simulink model "test4"  (R2015a)
settings: Solver=ode3  SolverMode=SingleTasking  StartTime=0.0  StopTime=10.0  RelTol=1e-3
libraries: simulink_extras x1, simulink x1
settings Model: ExtModeTrigDuration=2  Creator=kkhoo  LastModifiedBy=kkhoo
settings OptimizationCC: OptimizeModelRefInitCode=on  LifeSpan=1
settings DebuggingCC: UnderspecifiedInitializationDetection=Classic  MergeDetectMultiDrivingBlocksExec=none
settings HardwareCC: ProdBitPerInt=16  ProdBitPerPointer=8  ProdIntDivRoundTo=Zero  ProdEndianess=LittleEndian  ProdWordSize=8  ProdHWDeviceType=Atmel->AVR
settings RTWCC: SystemTargetFile=realtime.tlc  GenerateMakefile=off  TemplateMakefile=realtime.tmf  Description=Run on Target Hardware  RTWVerbose=off  CustomSource=src/Engduino.h src/engduino_wrappers.cpp
settings ERTTargetCC: CombineOutputUpdateFcns=off  ExtModeTransport=3  ExtModeMexFile=ext_serial_win32_comm_rtt  ExtModeMexArgs=0 1 9600  ERTSrcFileBannerTemplate=realtime_code_template.cgt  ERTHdrFileBannerTemplate=realtime_code_template.cgt  ERTDataSrcFileTemplate=realtime_code_template.cgt  ERTDataHdrFileTemplate=realtime_code_template.cgt  ERTCustomFileTemplate=realtime_file_process.tlc

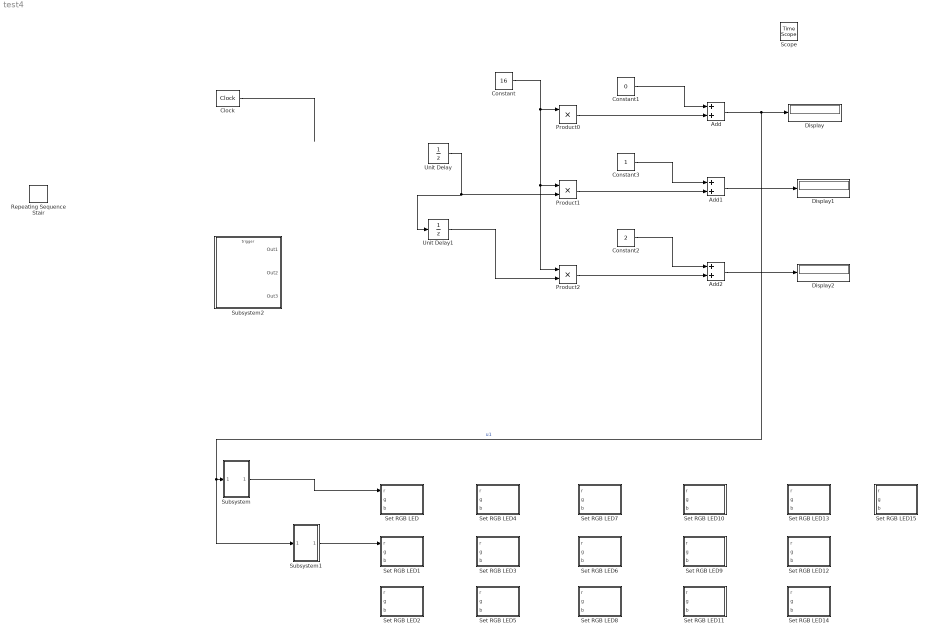
== system test4 ==
  Add : Sum  AccumDataTypeStr=single
  Add1 : Sum  AccumDataTypeStr=single
  Add2 : Sum  AccumDataTypeStr=single
  Clock : simulink_extras/Flip Flops/Clock  period=1000000
  Constant : Constant  Value=16  OutDataTypeStr=single
  Constant1 : Constant  Value=0  OutDataTypeStr=single
  Constant2 : Constant  Value=2  OutDataTypeStr=single
  Constant3 : Constant  OutDataTypeStr=single
  Display : Display
  Display1 : Display
  Display2 : Display
  "Product0 " : Product  OutDataTypeStr=single
  Product1 : Product  OutDataTypeStr=single
  Product2 : Product  OutDataTypeStr=single  InputSameDT=on
  Repeating Sequence Stair : simulink/Sources/Repeating Sequence Stair  OutValues=[0 1 2 3 4 5 6 7 8 9 10 11 12 13 14 15].'  tsamp=0.001  OutMin=[]  OutMax=[]  OutDataTypeStr=single  OutputDataTypeScalingMode=single  OutDataType=fixdt(0,8)  ConRadixGroup=Best Precision: Vector-wise  OutScaling=2^-12
  Scope : TimeScope
  Set RGB LED : MATLAB Function  LoadFcn=|  TreatAsAtomicUnit=on  mask(RGB LED){led_index=0}
      | set_param(gcs, 'CustomSource', strjoin(unique([strsplit(get_param(gcs, 'CustomSource')) ...
      |  'src/engduino_wrappers.cpp' 'src/Engduino.h'])));
      mask prompts: led_index "LED index"
      mask help:
      | Control the Red, Green and Blue color values of the LED specified by the LED index parameter.
      | Both the LED index and the three color values are of type uint8 and must be in the range 0-15.
      settings: AttributesFormatString=LED %<led_index>
  Set RGB LED1 : MATLAB Function  LoadFcn=|  TreatAsAtomicUnit=on  mask(RGB LED){led_index=1}
      | set_param(gcs, 'CustomSource', strjoin(unique([strsplit(get_param(gcs, 'CustomSource')) ...
      |  'src/engduino_wrappers.cpp' 'src/Engduino.h'])));
      mask prompts: led_index "LED index"
      mask help:
      | Control the Red, Green and Blue color values of the LED specified by the LED index parameter.
      | Both the LED index and the three color values are of type uint8 and must be in the range 0-15.
      settings: AttributesFormatString=LED %<led_index>
  Set RGB LED10 : MATLAB Function  LoadFcn=|  TreatAsAtomicUnit=on  mask(RGB LED){led_index=9}
      | set_param(gcs, 'CustomSource', strjoin(unique([strsplit(get_param(gcs, 'CustomSource')) ...
      |  'src/engduino_wrappers.cpp' 'src/Engduino.h'])));
      mask prompts: led_index "LED index"
      mask help:
      | Control the Red, Green and Blue color values of the LED specified by the LED index parameter.
      | Both the LED index and the three color values are of type uint8 and must be in the range 0-15.
      settings: AttributesFormatString=LED %<led_index>
  Set RGB LED11 : MATLAB Function  LoadFcn=|  TreatAsAtomicUnit=on  mask(RGB LED){led_index=11}
      | set_param(gcs, 'CustomSource', strjoin(unique([strsplit(get_param(gcs, 'CustomSource')) ...
      |  'src/engduino_wrappers.cpp' 'src/Engduino.h'])));
      mask prompts: led_index "LED index"
      mask help:
      | Control the Red, Green and Blue color values of the LED specified by the LED index parameter.
      | Both the LED index and the three color values are of type uint8 and must be in the range 0-15.
      settings: AttributesFormatString=LED %<led_index>
  Set RGB LED12 : MATLAB Function  LoadFcn=|  TreatAsAtomicUnit=on  mask(RGB LED){led_index=13}
      | set_param(gcs, 'CustomSource', strjoin(unique([strsplit(get_param(gcs, 'CustomSource')) ...
      |  'src/engduino_wrappers.cpp' 'src/Engduino.h'])));
      mask prompts: led_index "LED index"
      mask help:
      | Control the Red, Green and Blue color values of the LED specified by the LED index parameter.
      | Both the LED index and the three color values are of type uint8 and must be in the range 0-15.
      settings: AttributesFormatString=LED %<led_index>
  Set RGB LED13 : MATLAB Function  LoadFcn=|  TreatAsAtomicUnit=on  mask(RGB LED){led_index=12}
      | set_param(gcs, 'CustomSource', strjoin(unique([strsplit(get_param(gcs, 'CustomSource')) ...
      |  'src/engduino_wrappers.cpp' 'src/Engduino.h'])));
      mask prompts: led_index "LED index"
      mask help:
      | Control the Red, Green and Blue color values of the LED specified by the LED index parameter.
      | Both the LED index and the three color values are of type uint8 and must be in the range 0-15.
      settings: AttributesFormatString=LED %<led_index>
  Set RGB LED14 : MATLAB Function  LoadFcn=|  TreatAsAtomicUnit=on  mask(RGB LED){led_index=14}
      | set_param(gcs, 'CustomSource', strjoin(unique([strsplit(get_param(gcs, 'CustomSource')) ...
      |  'src/engduino_wrappers.cpp' 'src/Engduino.h'])));
      mask prompts: led_index "LED index"
      mask help:
      | Control the Red, Green and Blue color values of the LED specified by the LED index parameter.
      | Both the LED index and the three color values are of type uint8 and must be in the range 0-15.
      settings: AttributesFormatString=LED %<led_index>
  Set RGB LED15 : MATLAB Function  LoadFcn=|  TreatAsAtomicUnit=on  mask(RGB LED){led_index=15}
      | set_param(gcs, 'CustomSource', strjoin(unique([strsplit(get_param(gcs, 'CustomSource')) ...
      |  'src/engduino_wrappers.cpp' 'src/Engduino.h'])));
      mask prompts: led_index "LED index"
      mask help:
      | Control the Red, Green and Blue color values of the LED specified by the LED index parameter.
      | Both the LED index and the three color values are of type uint8 and must be in the range 0-15.
      settings: AttributesFormatString=LED %<led_index>
  Set RGB LED2 : MATLAB Function  LoadFcn=|  TreatAsAtomicUnit=on  mask(RGB LED){led_index=2}
      | set_param(gcs, 'CustomSource', strjoin(unique([strsplit(get_param(gcs, 'CustomSource')) ...
      |  'src/engduino_wrappers.cpp' 'src/Engduino.h'])));
      mask prompts: led_index "LED index"
      mask help:
      | Control the Red, Green and Blue color values of the LED specified by the LED index parameter.
      | Both the LED index and the three color values are of type uint8 and must be in the range 0-15.
      settings: AttributesFormatString=LED %<led_index>
  Set RGB LED3 : MATLAB Function  LoadFcn=|  TreatAsAtomicUnit=on  mask(RGB LED){led_index=4}
      | set_param(gcs, 'CustomSource', strjoin(unique([strsplit(get_param(gcs, 'CustomSource')) ...
      |  'src/engduino_wrappers.cpp' 'src/Engduino.h'])));
      mask prompts: led_index "LED index"
      mask help:
      | Control the Red, Green and Blue color values of the LED specified by the LED index parameter.
      | Both the LED index and the three color values are of type uint8 and must be in the range 0-15.
      settings: AttributesFormatString=LED %<led_index>
  Set RGB LED4 : MATLAB Function  LoadFcn=|  TreatAsAtomicUnit=on  mask(RGB LED){led_index=3}
      | set_param(gcs, 'CustomSource', strjoin(unique([strsplit(get_param(gcs, 'CustomSource')) ...
      |  'src/engduino_wrappers.cpp' 'src/Engduino.h'])));
      mask prompts: led_index "LED index"
      mask help:
      | Control the Red, Green and Blue color values of the LED specified by the LED index parameter.
      | Both the LED index and the three color values are of type uint8 and must be in the range 0-15.
      settings: AttributesFormatString=LED %<led_index>
  Set RGB LED5 : MATLAB Function  LoadFcn=|  TreatAsAtomicUnit=on  mask(RGB LED){led_index=5}
      | set_param(gcs, 'CustomSource', strjoin(unique([strsplit(get_param(gcs, 'CustomSource')) ...
      |  'src/engduino_wrappers.cpp' 'src/Engduino.h'])));
      mask prompts: led_index "LED index"
      mask help:
      | Control the Red, Green and Blue color values of the LED specified by the LED index parameter.
      | Both the LED index and the three color values are of type uint8 and must be in the range 0-15.
      settings: AttributesFormatString=LED %<led_index>
  Set RGB LED6 : MATLAB Function  LoadFcn=|  TreatAsAtomicUnit=on  mask(RGB LED){led_index=7}
      | set_param(gcs, 'CustomSource', strjoin(unique([strsplit(get_param(gcs, 'CustomSource')) ...
      |  'src/engduino_wrappers.cpp' 'src/Engduino.h'])));
      mask prompts: led_index "LED index"
      mask help:
      | Control the Red, Green and Blue color values of the LED specified by the LED index parameter.
      | Both the LED index and the three color values are of type uint8 and must be in the range 0-15.
      settings: AttributesFormatString=LED %<led_index>
  Set RGB LED7 : MATLAB Function  LoadFcn=|  TreatAsAtomicUnit=on  mask(RGB LED){led_index=6}
      | set_param(gcs, 'CustomSource', strjoin(unique([strsplit(get_param(gcs, 'CustomSource')) ...
      |  'src/engduino_wrappers.cpp' 'src/Engduino.h'])));
      mask prompts: led_index "LED index"
      mask help:
      | Control the Red, Green and Blue color values of the LED specified by the LED index parameter.
      | Both the LED index and the three color values are of type uint8 and must be in the range 0-15.
      settings: AttributesFormatString=LED %<led_index>
  Set RGB LED8 : MATLAB Function  LoadFcn=|  TreatAsAtomicUnit=on  mask(RGB LED){led_index=8}
      | set_param(gcs, 'CustomSource', strjoin(unique([strsplit(get_param(gcs, 'CustomSource')) ...
      |  'src/engduino_wrappers.cpp' 'src/Engduino.h'])));
      mask prompts: led_index "LED index"
      mask help:
      | Control the Red, Green and Blue color values of the LED specified by the LED index parameter.
      | Both the LED index and the three color values are of type uint8 and must be in the range 0-15.
      settings: AttributesFormatString=LED %<led_index>
  Set RGB LED9 : MATLAB Function  LoadFcn=|  TreatAsAtomicUnit=on  mask(RGB LED){led_index=10}
      | set_param(gcs, 'CustomSource', strjoin(unique([strsplit(get_param(gcs, 'CustomSource')) ...
      |  'src/engduino_wrappers.cpp' 'src/Engduino.h'])));
      mask prompts: led_index "LED index"
      mask help:
      | Control the Red, Green and Blue color values of the LED specified by the LED index parameter.
      | Both the LED index and the three color values are of type uint8 and must be in the range 0-15.
      settings: AttributesFormatString=LED %<led_index>
  Subsystem : Subsystem
  Subsystem1 : Subsystem
  Subsystem2 : Subsystem
  Unit Delay : UnitDelay  SampleTime=-1
  Unit Delay1 : UnitDelay  SampleTime=-1
  wires:
  Unit Delay/1 -> Unit Delay1/1, Product1/2
  Constant/1 -> "Product0 "/1, Product2/1, Product1/1
  Unit Delay1/1 -> Product2/2
  Constant1/1 -> Add/1
  "Product0 "/1 -> Add/2
  Constant3/1 -> Add1/1
  Product1/1 -> Add1/2
  Constant2/1 -> Add2/1
  Product2/1 -> Add2/2
  Add/1 -> Subsystem1/1(In1), Subsystem/1(In1), Display/1  "u1"
  Add1/1 -> Display1/1
  Add2/1 -> Display2/1
  Subsystem/1(Out1) -> Set RGB LED/1(r)
  Subsystem1/1(Out1) -> Set RGB LED1/1(r)
  ? -> Scope/1, "Product0 "/2, Unit Delay/1
  Clock/1 -> ?

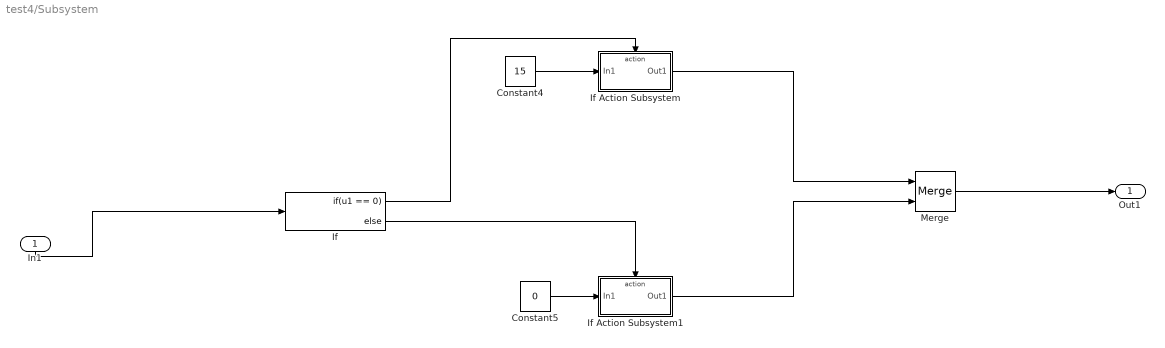
== system test4/Subsystem ==
  In1 : Inport
  Constant4 : Constant  Value=15  OutDataTypeStr=uint8
  Constant5 : Constant  Value=0  OutDataTypeStr=uint8
  If : If  IfExpression=u1 == 0
  If Action Subsystem : Subsystem  TreatAsAtomicUnit=on
  If Action Subsystem1 : Subsystem  TreatAsAtomicUnit=on
  Merge : Merge
  Out1 : Outport  OutDataTypeStr=uint8
  wires:
  If/1 -> If Action Subsystem/Action
  If/2 -> If Action Subsystem1/Action
  In1/1 -> If/1
  Constant5/1 -> If Action Subsystem1/1(In1)
  Merge/1 -> Out1/1
  Constant4/1 -> If Action Subsystem/1(In1)
  If Action Subsystem/1(Out1) -> Merge/1
  If Action Subsystem1/1(Out1) -> Merge/2

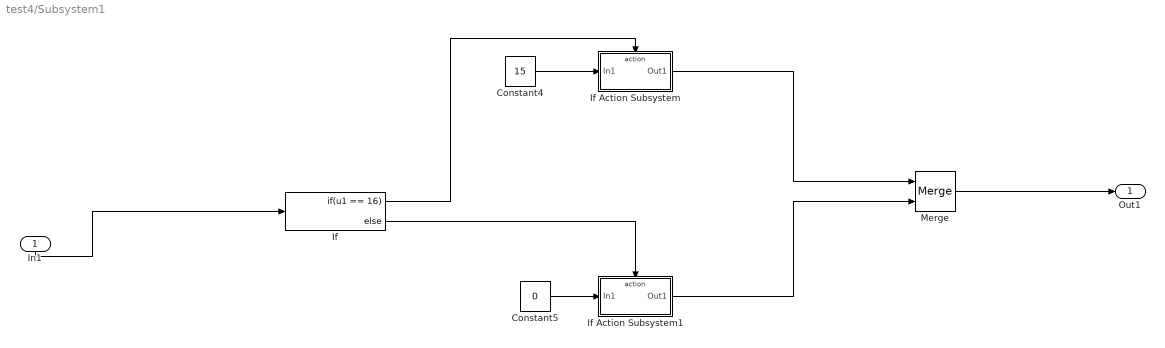
== system test4/Subsystem1 ==
  In1 : Inport
  Constant4 : Constant  Value=15  OutDataTypeStr=uint8
  Constant5 : Constant  Value=0  OutDataTypeStr=uint8
  If : If  IfExpression=u1 == 16
  If Action Subsystem : Subsystem  TreatAsAtomicUnit=on
  If Action Subsystem1 : Subsystem  TreatAsAtomicUnit=on
  Merge : Merge
  Out1 : Outport  OutDataTypeStr=uint8
  wires:
  If/1 -> If Action Subsystem/Action
  If/2 -> If Action Subsystem1/Action
  In1/1 -> If/1
  Constant5/1 -> If Action Subsystem1/1(In1)
  Merge/1 -> Out1/1
  Constant4/1 -> If Action Subsystem/1(In1)
  If Action Subsystem/1(Out1) -> Merge/1
  If Action Subsystem1/1(Out1) -> Merge/2

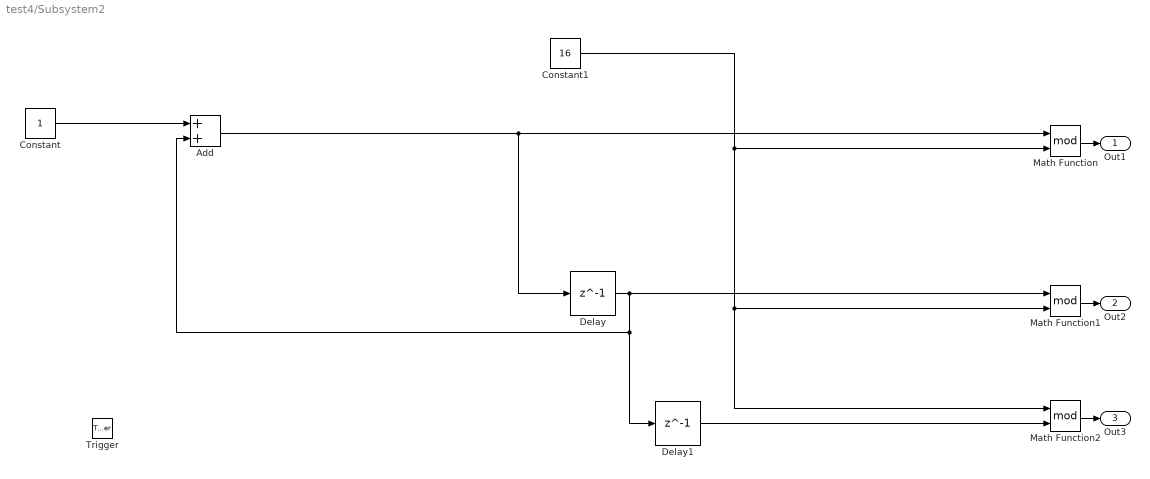
== system test4/Subsystem2 ==
  Trigger : TriggerPort  PortDimensions=1
  Add : Sum
  Constant : Constant
  Constant1 : Constant  Value=16
  Delay : Delay  DelayLength=1  InitialCondition=0
  Delay1 : Delay  DelayLength=1  InitialCondition=0
  Math Function : Math  Operator=mod  SaturateOnIntegerOverflow=on
  Math Function1 : Math  Operator=mod  SaturateOnIntegerOverflow=on
  Math Function2 : Math  Operator=mod  SaturateOnIntegerOverflow=on
  Out1 : Outport
  Out2 : Outport  Port=2
  Out3 : Outport  Port=3
  wires:
  Add/1 -> Math Function/1, Delay/1
  Constant/1 -> Add/1
  Math Function/1 -> Out1/1
  Math Function2/1 -> Out3/1
  Delay1/1 -> Math Function2/2
  Math Function1/1 -> Out2/1
  Constant1/1 -> Math Function/2, Math Function2/1, Math Function1/2
  Delay/1 -> Delay1/1, Add/2, Math Function1/1

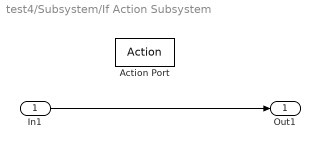
== system test4/Subsystem/If Action Subsystem ==
  In1 : Inport
  Action Port : ActionPort  ActionType=then
  Out1 : Outport  OutDataTypeStr=uint8
  wires:
  In1/1 -> Out1/1

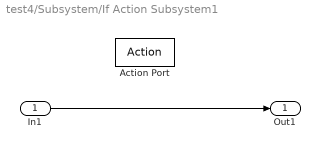
== system test4/Subsystem/If Action Subsystem1 ==
  In1 : Inport
  Action Port : ActionPort  ActionType=else
  Out1 : Outport  OutDataTypeStr=uint8
  wires:
  In1/1 -> Out1/1

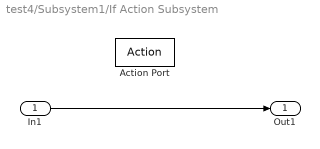
== system test4/Subsystem1/If Action Subsystem ==
  In1 : Inport
  Action Port : ActionPort  ActionType=then
  Out1 : Outport  OutDataTypeStr=uint8
  wires:
  In1/1 -> Out1/1

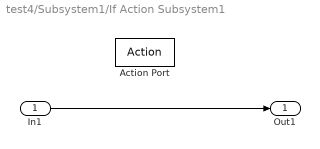
== system test4/Subsystem1/If Action Subsystem1 ==
  In1 : Inport
  Action Port : ActionPort  ActionType=else
  Out1 : Outport  OutDataTypeStr=uint8
  wires:
  In1/1 -> Out1/1

== matlab function test4/Set RGB LED2 ==
  data: led_index parameter uint8 [0..15]; r input uint8 [0..15]; g input uint8 [0..15]; b input uint8 [0..15]
function rgb_led(led_index, r, g, b)

if strcmp(coder.target, 'rtw')
    coder.ceval('rgb_leds_wrapper', led_index, r, g, b);
end

== matlab function test4/Set RGB LED3 ==
  data: led_index parameter uint8 [0..15]; r input uint8 [0..15]; g input uint8 [0..15]; b input uint8 [0..15]
function rgb_led(led_index, r, g, b)

if strcmp(coder.target, 'rtw')
    coder.ceval('rgb_leds_wrapper', led_index, r, g, b);
end

== matlab function test4/Set RGB LED ==
  data: led_index parameter uint8 [0..15]; r input uint8 [0..15]; g input uint8 [0..15]; b input uint8 [0..15]
function rgb_led(led_index, r, g, b)

if strcmp(coder.target, 'rtw')
    coder.ceval('rgb_leds_wrapper', led_index, r, g, b);
end

== matlab function test4/Set RGB LED1 ==
  data: led_index parameter uint8 [0..15]; r input uint8 [0..15]; g input uint8 [0..15]; b input uint8 [0..15]
function rgb_led(led_index, r, g, b)

if strcmp(coder.target, 'rtw')
    coder.ceval('rgb_leds_wrapper', led_index, r, g, b);
end

== matlab function test4/Set RGB LED4 ==
  data: led_index parameter uint8 [0..15]; r input uint8 [0..15]; g input uint8 [0..15]; b input uint8 [0..15]
function rgb_led(led_index, r, g, b)

if strcmp(coder.target, 'rtw')
    coder.ceval('rgb_leds_wrapper', led_index, r, g, b);
end

== matlab function test4/Set RGB LED5 ==
  data: led_index parameter uint8 [0..15]; r input uint8 [0..15]; g input uint8 [0..15]; b input uint8 [0..15]
function rgb_led(led_index, r, g, b)

if strcmp(coder.target, 'rtw')
    coder.ceval('rgb_leds_wrapper', led_index, r, g, b);
end

== matlab function test4/Set RGB LED6 ==
  data: led_index parameter uint8 [0..15]; r input uint8 [0..15]; g input uint8 [0..15]; b input uint8 [0..15]
function rgb_led(led_index, r, g, b)

if strcmp(coder.target, 'rtw')
    coder.ceval('rgb_leds_wrapper', led_index, r, g, b);
end

== matlab function test4/Set RGB LED7 ==
  data: led_index parameter uint8 [0..15]; r input uint8 [0..15]; g input uint8 [0..15]; b input uint8 [0..15]
function rgb_led(led_index, r, g, b)

if strcmp(coder.target, 'rtw')
    coder.ceval('rgb_leds_wrapper', led_index, r, g, b);
end

== matlab function test4/Set RGB LED8 ==
  data: led_index parameter uint8 [0..15]; r input uint8 [0..15]; g input uint8 [0..15]; b input uint8 [0..15]
function rgb_led(led_index, r, g, b)

if strcmp(coder.target, 'rtw')
    coder.ceval('rgb_leds_wrapper', led_index, r, g, b);
end

== matlab function test4/Set RGB LED10 ==
  data: led_index parameter uint8 [0..15]; r input uint8 [0..15]; g input uint8 [0..15]; b input uint8 [0..15]
function rgb_led(led_index, r, g, b)

if strcmp(coder.target, 'rtw')
    coder.ceval('rgb_leds_wrapper', led_index, r, g, b);
end

== matlab function test4/Set RGB LED11 ==
  data: led_index parameter uint8 [0..15]; r input uint8 [0..15]; g input uint8 [0..15]; b input uint8 [0..15]
function rgb_led(led_index, r, g, b)

if strcmp(coder.target, 'rtw')
    coder.ceval('rgb_leds_wrapper', led_index, r, g, b);
end

== matlab function test4/Set RGB LED9 ==
  data: led_index parameter uint8 [0..15]; r input uint8 [0..15]; g input uint8 [0..15]; b input uint8 [0..15]
function rgb_led(led_index, r, g, b)

if strcmp(coder.target, 'rtw')
    coder.ceval('rgb_leds_wrapper', led_index, r, g, b);
end

== matlab function test4/Set RGB LED12 ==
  data: led_index parameter uint8 [0..15]; r input uint8 [0..15]; g input uint8 [0..15]; b input uint8 [0..15]
function rgb_led(led_index, r, g, b)

if strcmp(coder.target, 'rtw')
    coder.ceval('rgb_leds_wrapper', led_index, r, g, b);
end

== matlab function test4/Set RGB LED13 ==
  data: led_index parameter uint8 [0..15]; r input uint8 [0..15]; g input uint8 [0..15]; b input uint8 [0..15]
function rgb_led(led_index, r, g, b)

if strcmp(coder.target, 'rtw')
    coder.ceval('rgb_leds_wrapper', led_index, r, g, b);
end

== matlab function test4/Set RGB LED14 ==
  data: led_index parameter uint8 [0..15]; r input uint8 [0..15]; g input uint8 [0..15]; b input uint8 [0..15]
function rgb_led(led_index, r, g, b)

if strcmp(coder.target, 'rtw')
    coder.ceval('rgb_leds_wrapper', led_index, r, g, b);
end

== matlab function test4/Set RGB LED15 ==
  data: led_index parameter uint8 [0..15]; r input uint8 [0..15]; g input uint8 [0..15]; b input uint8 [0..15]
function rgb_led(led_index, r, g, b)

if strcmp(coder.target, 'rtw')
    coder.ceval('rgb_leds_wrapper', led_index, r, g, b);
end
